simulink model "unknown"  (R2022b)
settings: Solver=VariableStepAuto  StartTime=0.0  StopTime=50  RelTol=1e-3
libraries: dsparch4 x3, simulink x1, dspfdesign x1, dspstat3 x1
settings Model: Creator=Lisa  LastModifiedBy=Lisa

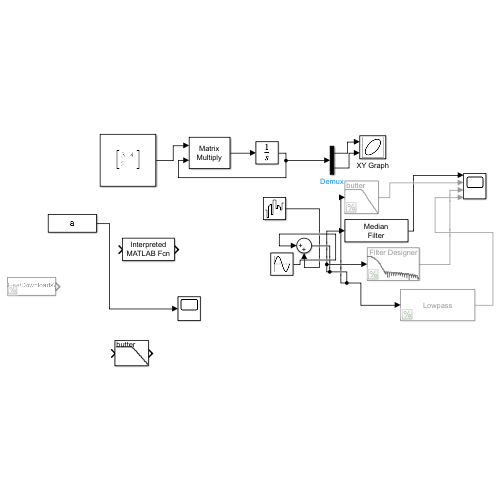
[thumbnail: Simulink's stored preview of the top-level diagram]
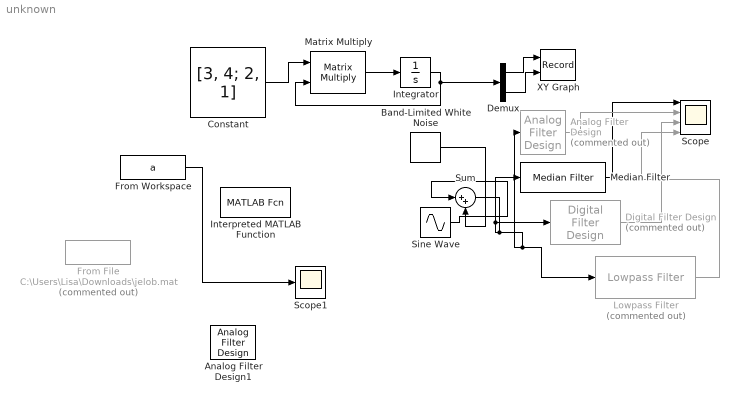
== system unknown ==
  Analog Filter Design : dsparch4/Analog Filter Design  Commented=on  method=Butterworth  filttype=Lowpass  N=8  Wlo=2  Whi=80  Rp=2  Rs=40
  Analog Filter Design1 : dsparch4/Analog Filter Design  method=Butterworth  filttype=Lowpass  N=8  Wlo=30  Whi=80  Rp=2  Rs=40
  Band-Limited White Noise : simulink/Sources/Band-Limited White Noise  Cov=[0.1]  Ts=0.1  seed=[23341]
  Constant : Constant  Value=[3, 4; 2, 1]
  Demux : Demux  Outputs=2
  Digital Filter Design : dsparch4/Digital Filter Design  Commented=on  mwdsp_browser_bugfix_var=off
  From Workspace : FromWorkspace  VariableName=a  SampleTime=-1
  From File : FromFile  Commented=on  FileName=C:\Users\Lisa\Downloads\jelob.mat  SampleTime=1  ExtrapolationBeforeFirstDataPoint=Ground value
  Integrator : Integrator  InitialCondition=[1;20]
  Interpreted MATLAB Function : MATLABFcn
  Lowpass Filter : dspfdesign/Lowpass Filter  Commented=on  FilterType=FIR  DesignForMinimumOrder=on  FilterOrder=50  PassbandFrequency=1e3  StopbandFrequency=4e3  PassbandRipple=0.7  StopbandAttenuation=150  InheritSampleRate=off  SampleRate=45600  SimulateUsing=Interpreted execution  roundingMode=Floor  coeffsDataTypeStr=fixdt(1,16)
  Matrix Multiply : Product  Multiplication=Matrix(*)
  Median Filter : dspstat3/Median Filter  WindowLength=205  SimulateUsing=Interpreted execution
      settings: LibrarySourceBlock=|
      | dspfdesign/Median
      | Filter
  Scope : Scope  NumInputPorts=4
  Scope1 : Scope
  Sine Wave : Sin  SampleTime=0
  Sum : Sum  Inputs=|++
  XY Graph : Record  FileSettingsInternal="{\"entries\":[{\"content\":{\"excelSettings\":{\"content\":{},\"type\":\"Streamout.ExcelSettings\"}},\"type\":\"Streamout.FileSettingStorage\",\"uuid\":\"9de67a92-066e-4da0-aff2-1a59f583883a\"}],\"packageUris\":[\"http://schema.mathworks.com/mf0/streamout_blocks/R2020a\"],\"version\":\"1.0\"}"  Layout=[1 1]  SignalsInternal="{\"entries\":[{\"content\":{\"signals\":[{\"content\":{\"blockPath\":[\"untitled/XY Graph\"],\"channel\":[],\"dimensions\":[1],\"domain\":\"untitled/XY Graph\",\"lineColor\":\"#a2142f\",\"plots\":[1],\"port\":1,\"sid\":[\"\"],\"signalID\":1010,\"signalName\":\"Demux:1\"},\"type\":\"RecordBlkView.Signal\",\"uuid\":\"ef06d7a2-61bb-42cb-a983-6de5cfa2bbe5\"},{\"content\":{\"blockPath\":[\"untitled/XY Graph\"],\"channel\":[],\"dimensions\":[1],\"domain\":\"untitled/XY Graph\",\"lineColor\":\"#139fff\",\"plots\":[1],\"port\":2,\"sid\":[\"\"],\"signalID\":1014,\"signalName\":\"Demux:2\"},\"type\":\"RecordBlkView.Signal\",\"uuid\":\"94d4e86d-aea0-4d97-a0d7-cd9f9259e5a4\"}]},\"type\":\"RecordBlkView.InputSignals\",\"uuid\":\"a111ad5c-d54e-4436-8e5a-d800f0b4b673\"}],\"packageUris\":[\"http://schema.mathworks.com/mf0/streamout_blocks/R2020a\"],\"version\":\"1.0\"}"  VisualizationBindings="{\"xyplotplugin\":{\"info\":[{\"series\":[{\"bindingParametersList\":[{\"parameter\":\"X-Axis\",\"signalID\":1010,\"signalName\":\"Demux:1\"},{\"parameter\":\"Y-Axis\",\"signalID\":1014,\"signalName\":\"Demux:2\"}],\"seriesID\":5364}],\"subplotID\":1}]}}"  CompatibilityTag=XY
  wires:
  Matrix Multiply/1 -> Integrator/1
  Constant/1 -> Matrix Multiply/1
  Integrator/1 -> Matrix Multiply/2, Demux/1
  Sine Wave/1 -> Sum/1
  Band-Limited White Noise/1 -> Sum/2
  Sum/1 -> Median Filter/1, Digital Filter Design/1, Analog Filter Design/1, Lowpass Filter/1
  Digital Filter Design/1 -> Scope/3
  Median Filter/1 -> Scope/1
  Analog Filter Design/1 -> Scope/2
  Demux/1 -> XY Graph/1
  Demux/2 -> XY Graph/2
  Lowpass Filter/1 -> Scope/4
  From Workspace/1 -> Scope1/1
